simulink model "modelS"  (R2018a)
settings: Solver=FixedStepAuto  StartTime=0.0  StopTime=2096.5202176570892  FixedStep=1e-3  RelTol=1e-6  EnableMultiTasking=on
model workspace (MAT data in the model file):
  modelS_spesession : sldodialogs.data.SessionData (value not decoded)
values from neighbouring files (symbols this model uses):
  a1 = 0.1125    [data_plotting.m]    (also in optim_fmincon.m; optim_ga.m; optim_ps.m; prepareDataSimulink.m)
  a2 = -0.1125    [data_plotting.m]    (also in optim_fmincon.m; optim_ga.m; optim_ps.m; prepareDataSimulink.m)
  a3 = -0.1125    [data_plotting.m]    (also in optim_fmincon.m; optim_ga.m; optim_ps.m; prepareDataSimulink.m)
  a4 = 0.1125    [data_plotting.m]    (also in optim_fmincon.m; optim_ga.m; optim_ps.m; prepareDataSimulink.m)
  b1 = 0.1125    [data_plotting.m]    (also in optim_fmincon.m; optim_ga.m; optim_ps.m; prepareDataSimulink.m)
  b2 = 0.1125    [data_plotting.m]    (also in optim_fmincon.m; optim_ga.m; optim_ps.m; prepareDataSimulink.m)
  b3 = -0.1125    [data_plotting.m]    (also in optim_fmincon.m; optim_ga.m; optim_ps.m; prepareDataSimulink.m)
  b4 = -0.1125    [data_plotting.m]    (also in optim_fmincon.m; optim_ga.m; optim_ps.m; prepareDataSimulink.m)
  r1 = 0.0254    [data_plotting.m]    (also in optim_fmincon.m; optim_ga.m; optim_ps.m; prepareDataSimulink.m)
  r2 = 0.0254    [data_plotting.m]    (also in optim_fmincon.m; optim_ga.m; optim_ps.m; prepareDataSimulink.m)
  r3 = 0.0254    [data_plotting.m]    (also in optim_fmincon.m; optim_ga.m; optim_ps.m; prepareDataSimulink.m)
  r4 = 0.0254    [data_plotting.m]    (also in optim_fmincon.m; optim_ga.m; optim_ps.m; prepareDataSimulink.m)
  T = 1e-3    (= 0.001)    [prepareDataSimulink.m]
undefined symbols (not defined in the file or in its folder): DiscIntNeverNeededParam
settings Model: Creator=jakov  LastModifiedBy=jakov
settings SolverCC: ZeroCrossAlgorithm=Adaptive  AlgebraicLoopSolver=LineSearch
settings DataIOCC: Decimation=10  ExternalInput=[x]  ReturnWorkspaceOutputs=on  OutputOption=AdditionalOutputTimes  OutputTimes=SDO_OutputTimes  ReturnWorkspaceOutputsName=SDOSimTest_Log
settings DebuggingCC: MaxConsecutiveZCsMsg=none

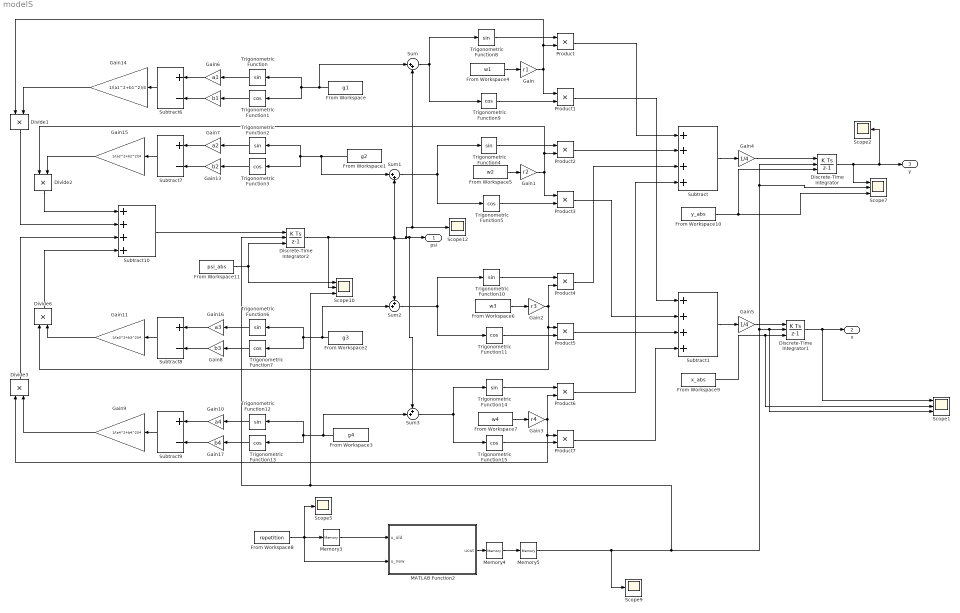
== system modelS ==
  " " : Gain  Gain=b1
  Discrete-Time Integrator : DiscreteIntegrator  ExternalReset=falling  InitialConditionSource=external  SampleTime=1e-3  ICPrevOutput=DiscIntNeverNeededParam  ICPrevScaledInput=DiscIntNeverNeededParam
  Discrete-Time Integrator1 : DiscreteIntegrator  ExternalReset=falling  InitialConditionSource=external  SampleTime=1e-3  ICPrevOutput=DiscIntNeverNeededParam  ICPrevScaledInput=DiscIntNeverNeededParam
  Discrete-Time Integrator2 : DiscreteIntegrator  ExternalReset=falling  InitialConditionSource=external  SampleTime=1e-3  ICPrevOutput=DiscIntNeverNeededParam  ICPrevScaledInput=DiscIntNeverNeededParam
  Divide{1..3,6} (4 alike) : Product  Inputs=**
  From Workspace : FromWorkspace  VariableName=g1  SampleTime=T
  From Workspace1 : FromWorkspace  VariableName=g2  SampleTime=T
  From Workspace10 : FromWorkspace  VariableName=y_abs  SampleTime=0
  From Workspace11 : FromWorkspace  VariableName=psi_abs  SampleTime=T
  From Workspace2 : FromWorkspace  VariableName=g3  SampleTime=T
  From Workspace3 : FromWorkspace  VariableName=g4  SampleTime=T
  From Workspace4 : FromWorkspace  VariableName=w1  SampleTime=T
  From Workspace5 : FromWorkspace  VariableName=w2  SampleTime=T
  From Workspace6 : FromWorkspace  VariableName=w3  SampleTime=T
  From Workspace7 : FromWorkspace  VariableName=w4  SampleTime=T
  From Workspace8 : FromWorkspace  VariableName=repetition  OutDataTypeStr=double  SampleTime=T
  From Workspace9 : FromWorkspace  VariableName=x_abs  SampleTime=T
  Gain : Gain  Gain=r1
  Gain1 : Gain  Gain=r2
  Gain10 : Gain  Gain=a4
  Gain11 : Gain  Gain=1/(a3^2+b3^2)/4
  Gain13 : Gain  Gain=b2
  Gain14 : Gain  Gain=1/(a1^2+b1^2)/4
  Gain15 : Gain  Gain=1/(a2^2+b2^2)/4
  Gain16 : Gain  Gain=a3
  Gain17 : Gain  Gain=b4
  Gain2 : Gain  Gain=r3
  Gain3 : Gain  Gain=r4
  Gain4 : Gain  Gain=1/4
  Gain5 : Gain  Gain=1/4
  Gain6 : Gain  Gain=a1
  Gain7 : Gain  Gain=a2
  Gain8 : Gain  Gain=b3
  Gain9 : Gain  Gain=1/(a4^2+b4^2)/4
  MATLAB Function2 : MATLAB Function  TreatAsAtomicUnit=on
  Memory3 : Memory  LinearizeAsDelay=on
  Memory4 : Memory  LinearizeAsDelay=on
  Memory5 : Memory  LinearizeAsDelay=on
  Product{,1..7} (8 alike) : Product
  Scope1 : Scope  NumInputPorts=3
  Scope10 : Scope  NumInputPorts=3
  Scope{2,5,9,12} (4 alike) : Scope
  Scope7 : Scope  NumInputPorts=3
  Subtract : Sum  Inputs=++++
  Subtract1 : Sum  Inputs=++++
  Subtract10 : Sum  Inputs=++++
  Subtract{6..9} (4 alike) : Sum  Inputs=+-
  Sum : Sum  Inputs=|++
  Sum1 : Sum  Inputs=|++
  Sum2 : Sum  Inputs=++|
  Sum3 : Sum  Inputs=++|
  Trigonometric Function{,2,4,6,8,10,12,14} (8 alike) : Trigonometry
  Trigonometric Function{1,3,5,7,9,11,13,15} (8 alike) : Trigonometry  Operator=cos
  "psi " : Outport  SampleTime=T
  x : Outport  Port=2  SampleTime=T
  y : Outport  Port=3  SampleTime=T
  wires:
  From Workspace/1 -> Sum/1, Trigonometric Function/1, Trigonometric Function1/1
  From Workspace4/1 -> Gain/1
  Sum/1 -> Trigonometric Function9/1, Trigonometric Function8/1
  Gain/1 -> Divide1/1, Product/2, Product1/1
  Trigonometric Function9/1 -> Product1/2
  Trigonometric Function8/1 -> Product/1
  Gain1/1 -> Divide2/1, Product2/2, Product3/1
  From Workspace5/1 -> Gain1/1
  Sum1/1 -> Trigonometric Function5/1, Trigonometric Function4/1
  Trigonometric Function4/1 -> Product2/1
  Trigonometric Function5/1 -> Product3/2
  Gain2/1 -> Product4/2, Divide6/1, Product5/1
  From Workspace6/1 -> Gain2/1
  Sum2/1 -> Trigonometric Function10/1, Trigonometric Function11/1
  Trigonometric Function10/1 -> Product4/1
  Trigonometric Function11/1 -> Product5/2
  Gain3/1 -> Product7/1, Divide3/1, Product6/2
  From Workspace7/1 -> Gain3/1
  Sum3/1 -> Trigonometric Function15/1, Trigonometric Function14/1
  Trigonometric Function14/1 -> Product6/1
  Trigonometric Function15/1 -> Product7/2
  Product/1 -> Subtract/1
  Product2/1 -> Subtract/2
  Product4/1 -> Subtract/3
  Product6/1 -> Subtract/4
  Product7/1 -> Subtract1/4
  Product5/1 -> Subtract1/3
  Product3/1 -> Subtract1/2
  Product1/1 -> Subtract1/1
  Subtract1/1 -> Gain5/1
  Subtract/1 -> Gain4/1
  Trigonometric Function/1 -> Gain6/1
  Trigonometric Function1/1 -> " "/1
  Gain6/1 -> Subtract6/1
  " "/1 -> Subtract6/2
  Subtract6/1 -> Gain14/1
  Gain7/1 -> Subtract7/1
  Subtract7/1 -> Gain15/1
  From Workspace1/1 -> Trigonometric Function2/1, Trigonometric Function3/1, Sum1/1
  Gain13/1 -> Subtract7/2
  Trigonometric Function3/1 -> Gain13/1
  Trigonometric Function2/1 -> Gain7/1
  Trigonometric Function6/1 -> Gain16/1
  Trigonometric Function7/1 -> Gain8/1
  Gain16/1 -> Subtract8/1
  Gain8/1 -> Subtract8/2
  From Workspace2/1 -> Trigonometric Function7/1, Trigonometric Function6/1, Sum2/2
  Trigonometric Function12/1 -> Gain10/1
  Trigonometric Function13/1 -> Gain17/1
  Gain17/1 -> Subtract9/2
  From Workspace3/1 -> Sum3/2, Trigonometric Function12/1, Trigonometric Function13/1
  Gain10/1 -> Subtract9/1
  Subtract9/1 -> Gain9/1
  Gain9/1 -> Divide3/2
  Subtract8/1 -> Gain11/1
  Gain11/1 -> Divide6/2
  Gain14/1 -> Divide1/2
  Gain15/1 -> Divide2/2
  Divide3/1 -> Subtract10/3
  Divide6/1 -> Subtract10/4
  Divide2/1 -> Subtract10/1
  Divide1/1 -> Subtract10/2
  MATLAB Function2/1(uout) -> Memory4/1
  From Workspace9/1 -> Discrete-Time Integrator1/3, Scope1/2
  From Workspace10/1 -> Discrete-Time Integrator/3, Scope7/3
  Subtract10/1 -> Discrete-Time Integrator2/1
  From Workspace11/1 -> Scope10/1, Discrete-Time Integrator2/3
  From Workspace8/1 -> MATLAB Function2/2(u_new), Memory3/1, Scope5/1
  Memory3/1 -> MATLAB Function2/1(u_old)
  Memory4/1 -> Memory5/1
  Memory5/1 -> Discrete-Time Integrator2/2, Scope10/3, Discrete-Time Integrator/2, Scope7/2, Discrete-Time Integrator1/2, Scope1/3, Scope9/1
  Discrete-Time Integrator2/1 -> Scope10/2, Sum2/1, Sum/2, Scope12/1, Sum3/1, "psi "/1, Sum1/2
  Gain4/1 -> Discrete-Time Integrator/1
  Discrete-Time Integrator/1 -> Scope2/1, y/1, Scope7/1
  Gain5/1 -> Discrete-Time Integrator1/1
  Discrete-Time Integrator1/1 -> Scope1/1, x/1

== matlab function modelS/MATLAB Function2 ==
  data: u_old input; uout output; u_new input
function uout  = change_repetition(u_old,u_new)
    uout=0;
    if(u_new~=u_old)
        uout=1;
    end
end
